simulink model "commviterbihdl7"  (R2020b)
settings: Solver=FixedStepDiscrete  StartTime=0.0  StopTime=5000  RelTol=1e-3
InitFcn:
  | EbNo=8;
libraries: commcnvcod2 x4, commdigbbndpm3 x4, dspquant2 x2, commchan3 x2, commsink2 x2, commrandsrc2 x1, commblksprivate x1
Description:
  | Viterbi Decoder Using Simulink(R) Blocks
  | This model shows how to use HDL Coder(TM) to check, generate,
  | and verify HDL for a fixed-point Viterbi decoder model built using Simulink(R) blocks.
settings Model: ExtModeAutoUpdateStatusClock=off  Creator=The MathWorks Inc.  LastModifiedBy=jeldo
settings DataIOCC: LimitDataPoints=on  SaveFormat=Array  SaveOutput=off  SignalLogging=off  SaveTime=off  ReturnWorkspaceOutputs=off
settings OptimizationCC: BlockReduction=off  ConditionallyExecuteInputs=off  DefaultParameterBehavior=Inlined  ExpressionDepthLimit=2147483647  InitFltsAndDblsToZero=on  EfficientMapNaN2IntZero=off  LifeSpan=inf
settings DebuggingCC: AlgebraicLoopMsg=error  UnderspecifiedInitializationDetection=Classic  MergeDetectMultiDrivingBlocksExec=none  SignalResolutionControl=TryResolveAllWithWarning  SolverPrmCheckMsg=warning  MultiTaskDSMMsg=warning  MultiTaskCondExecSysMsg=none  SingleTaskRateTransMsg=error  IntegerOverflowMsg=none  ParameterPrecisionLossMsg=none  FcnCallInpInsideContextMsg=warning  StateNameClashWarn=warning  SFUnexpectedBacktrackingDiag=warning  SFNoUnconditionalDefaultTransitionDiag=warning  SFExecutionAtInitializationDiag=none  IntegerSaturationMsg=none  ArithmeticOperatorsInVariantConditions=warning
settings HardwareCC: ProdBitPerPointer=32  ProdBitPerSizeT=32  ProdBitPerPtrDiffT=32  ProdLargestAtomicFloat=None  ProdIntDivRoundTo=Undefined  ProdEndianess=Unspecified  ProdWordSize=32  ProdHWDeviceType=ASIC/FPGA  ProdEqTarget=off
settings ModelReferenceCC: PropagateSignalLabelsOutOfModel=off
settings SFSimCC: SimUseLocalCustomCode=off  CustomCodeUndefinedFunction=UseInterfaceOnly
settings RTWCC: RTWUseLocalCustomCode=off
settings CodeAppCC: StateflowObjectComments=on
settings GRTTargetCC: TargetLangStandard=C89/C90 (ANSI)  CombineOutputUpdateFcns=off  GRTInterface=on
settings ConfigComp: CovMetricSettings=dw  CovSaveCumulativeToWorkspaceVar=on  CovSaveSingleToWorkspaceVar=on  CovExternalEMLEnable=off  CovSFcnEnable=off

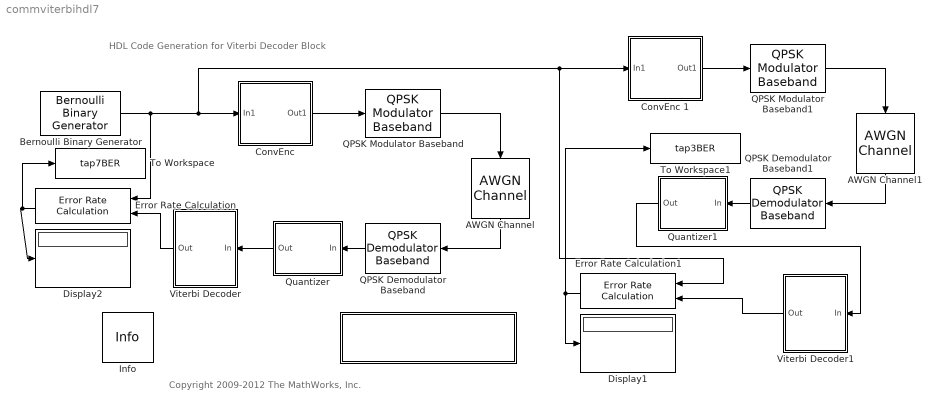
== system commviterbihdl7 ==
  note: Copyright 2009-2012 The MathWorks, Inc.
  note: HDL Code Generation for Viterbi Decoder Block
  " " : Subsystem
      settings: OpenFcn=hdldialog(bdroot)
      mask Display: disp('Launch HDL Dialog')
  " Quantizer" : Subsystem
  " Quantizer1" : Subsystem
  AWGN Channel : commchan3/AWGN Channel  InputProcessing=Columns as channels (frame based)  seed=123456  noiseMode="Signal to noise ratio  (Eb/No)"  EbNodB=EbNo+10*log10(1/2)  EsNodB=EsNo  SNRdB=10  bitsPerSym=2  Ps=1  Tsym=1  variance=1
  AWGN Channel1 : commchan3/AWGN Channel  InputProcessing=Columns as channels (frame based)  seed=123456  noiseMode="Signal to noise ratio  (Eb/No)"  EbNodB=EbNo+10*log10(1/2)  EsNodB=EsNo  SNRdB=10  bitsPerSym=2  Ps=1  Tsym=2  variance=1
  Bernoulli Binary Generator : commrandsrc2/Bernoulli Binary Generator  P=0.5  seed=610  Ts=1  frameBased=off  sampPerFrame=1  orient=off  outDataType=boolean
      settings: SourceProductBaseCode=CM
  "ConvEnc " : Subsystem
  ConvEnc 1 : Subsystem
  Display1 : Display
  Display2 : Display
  Error Rate Calculation : commsink2/Error Rate Calculation  N=32  st_delay=0  cp_mode=Entire frame  subframe=[]  PMode=Port  WsName=BER_Data  RsMode2=off  stop=on  numErr=500  maxBits=1e6
  Error Rate Calculation1 : commsink2/Error Rate Calculation  N=32  st_delay=0  cp_mode=Entire frame  subframe=[]  PMode=Port  WsName=BER_Data  RsMode2=off  stop=off  numErr=500  maxBits=1e6
  Info : commblksprivate/Info  SystemSampleTime=-1  VariantActivationTime=update diagram  Latency=0  AutoFrameSizeCalculation=off
      settings: SourceProductBaseCode=CM
  QPSK Demodulator Baseband : commdigbbndpm3/QPSK Demodulator Baseband  OutType=Bit  DecType=Log-likelihood ratio  VarSource=Dialog  Variance=10^(-0.1*EbNo)  Dec=Gray  Ph=pi/4  outDtype1=Inherit via internal rule  outDtype2=Inherit via internal rule  derotateFactorWordLen=16  derotateFactorDataTypeStr=Inherit: Same word length as input  derotateFactorLastDataTypeStr=Inherit: Same word length as input
  QPSK Demodulator Baseband1 : commdigbbndpm3/QPSK Demodulator Baseband  OutType=Bit  DecType=Log-likelihood ratio  VarSource=Dialog  Variance=10^(-0.1*EbNo)  Dec=Gray  Ph=pi/4  outDtype1=Inherit via internal rule  outDtype2=Inherit via internal rule  derotateFactorWordLen=16  derotateFactorDataTypeStr=Inherit: Same word length as input  derotateFactorLastDataTypeStr=Inherit: Same word length as input
  QPSK Modulator Baseband : commdigbbndpm3/QPSK Modulator Baseband  InType=Bit  Enc=Gray  Ph=pi/4  outDtype=double  outWordLen=16  outUDDataType=sfix(16)  outFracLenMode=Best precision  outFracLen=15  outDataTypeStr=double  outLastDataTypeStr=double
  QPSK Modulator Baseband1 : commdigbbndpm3/QPSK Modulator Baseband  InType=Bit  Enc=Gray  Ph=pi/4  outDtype=double  outWordLen=16  outUDDataType=sfix(16)  outFracLenMode=Best precision  outFracLen=15  outDataTypeStr=double  outLastDataTypeStr=double
  To Workspace : ToWorkspace  VariableName=tap7BER  SaveFormat=Timeseries  SampleTime=-1
  To Workspace1 : ToWorkspace  VariableName=tap3BER  SaveFormat=Timeseries  SampleTime=-1
  Viterbi Decoder : Subsystem
  Viterbi Decoder1 : Subsystem
  wires:
  Error Rate Calculation/1 -> To Workspace/1, Display2/1
  " Quantizer"/1(Out) -> Viterbi Decoder/1(In)
  QPSK Modulator Baseband/1 -> AWGN Channel/1
  AWGN Channel/1 -> QPSK Demodulator Baseband/1
  QPSK Demodulator Baseband/1 -> " Quantizer"/1(In)
  Viterbi Decoder/1(Out) -> Error Rate Calculation/2
  "ConvEnc "/1(Out1) -> QPSK Modulator Baseband/1
  QPSK Modulator Baseband1/1 -> AWGN Channel1/1
  AWGN Channel1/1 -> QPSK Demodulator Baseband1/1
  QPSK Demodulator Baseband1/1 -> " Quantizer1"/1(In)
  Error Rate Calculation1/1 -> Display1/1, To Workspace1/1
  Bernoulli Binary Generator/1 -> ConvEnc 1/1(In1), Error Rate Calculation1/1, "ConvEnc "/1(In1), Error Rate Calculation/1
  " Quantizer1"/1(Out) -> Viterbi Decoder1/1(In)
  ConvEnc 1/1(Out1) -> QPSK Modulator Baseband1/1
  Viterbi Decoder1/1(Out) -> Error Rate Calculation1/2

== system commviterbihdl7/  ==

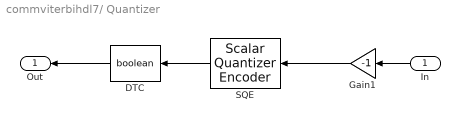
== system commviterbihdl7/ Quantizer ==
  In : Inport
  DTC : DataTypeConversion  OutDataTypeStr=boolean
  Gain1 : Gain  Gain=-1
  SQE : dspquant2/Scalar Quantizer Encoder  paramSrc=Specify via dialog  partType=Unbounded  BBoundary=[-6:2:6]/4  UBoundary=[-3:3]  SearchMethod=Linear  tieBreakRule=Choose the higher index  outQU=off  outQError=off  codebook=[1.5:9.5]  outStatus=off  invalidin=Clip  idtype=uint8  roundingMode=Floor  overflowMode=off
      settings: SourceProductBaseCode=DS
  Out : Outport
  wires:
  DTC/1 -> Out/1
  SQE/1 -> DTC/1
  Gain1/1 -> SQE/1
  In/1 -> Gain1/1

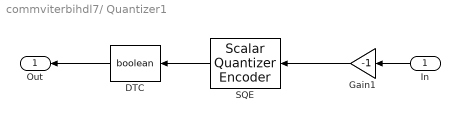
== system commviterbihdl7/ Quantizer1 ==
  In : Inport
  DTC : DataTypeConversion  OutDataTypeStr=boolean
  Gain1 : Gain  Gain=-1
  SQE : dspquant2/Scalar Quantizer Encoder  paramSrc=Specify via dialog  partType=Unbounded  BBoundary=[-6:2:6]/4  UBoundary=[-3:3]  SearchMethod=Linear  tieBreakRule=Choose the higher index  outQU=off  outQError=off  codebook=[1.5:9.5]  outStatus=off  invalidin=Clip  idtype=uint8  roundingMode=Floor  overflowMode=off
      settings: SourceProductBaseCode=DS
  Out : Outport
  wires:
  DTC/1 -> Out/1
  SQE/1 -> DTC/1
  Gain1/1 -> SQE/1
  In/1 -> Gain1/1

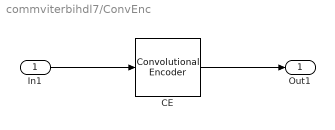
== system commviterbihdl7/ConvEnc  ==
  In1 : Inport
  CE : commcnvcod2/Convolutional Encoder  trellis=poly2trellis(7,[171 133])  opMode=Continuous  DelayedResetAction=off  hasIniStPort=off  hasFinStPort=off  usePuncVector=off  punctureVector=[1; 1; 0; 1; 0; 1]  reset=Unused parameter value
      settings: SourceProductBaseCode=CM
  Out1 : Outport
  wires:
  CE/1 -> Out1/1
  In1/1 -> CE/1

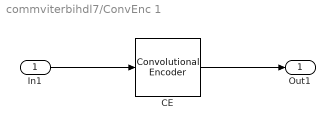
== system commviterbihdl7/ConvEnc 1 ==
  In1 : Inport
  CE : commcnvcod2/Convolutional Encoder  trellis=poly2trellis(3,[6 7])  opMode=Continuous  DelayedResetAction=off  hasIniStPort=off  hasFinStPort=off  usePuncVector=off  punctureVector=[1; 1; 0; 1; 0; 1]  reset=Unused parameter value
      settings: SourceProductBaseCode=CM
  Out1 : Outport
  wires:
  CE/1 -> Out1/1
  In1/1 -> CE/1

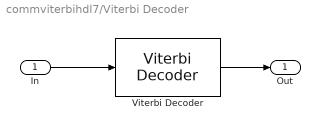
== system commviterbihdl7/Viterbi Decoder ==
  In : Inport
  Viterbi Decoder : commcnvcod2/Viterbi Decoder  trellis=poly2trellis(7,[171 133])  isPunctured=off  punctureVector=[1; 1; 0; 1; 0; 1]  erasures=off  dectype=Hard decision  nsdecb=3  runSigValErrCheck=off  tbdepth=32  opmode=Continuous  reset=off  delayedResetAction=off  smWordLength=16  outDataType=boolean
      settings: SourceProductBaseCode=CM
  Out : Outport
  wires:
  In/1 -> Viterbi Decoder/1
  Viterbi Decoder/1 -> Out/1

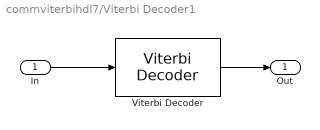
== system commviterbihdl7/Viterbi Decoder1 ==
  In : Inport
  Viterbi Decoder : commcnvcod2/Viterbi Decoder  trellis=poly2trellis(3,[6 7])  isPunctured=off  punctureVector=[1; 1; 0; 1; 0; 1]  erasures=off  dectype=Hard decision  nsdecb=3  runSigValErrCheck=off  tbdepth=32  opmode=Continuous  reset=off  delayedResetAction=off  smWordLength=16  outDataType=boolean
      settings: SourceProductBaseCode=CM
  Out : Outport
  wires:
  In/1 -> Viterbi Decoder/1
  Viterbi Decoder/1 -> Out/1
